simulink library "lib_dGrid"  (R2023b)
settings: Solver=VariableStepAuto  StartTime=0.0  StopTime=10.0  RelTol=1e-3
values from neighbouring files (symbols this model uses):
  C_PM = 10e-3    (= 0.01)    [my_MMC_param.m]
  Cbase = 1/Zbase/wb    (= 3.10849498226e-05)    [my_MMC_param.m]
  f0 = 50/fb    (= 1)    [my_MMC_param.m]
  Fn_filter = 1000    [my_MMC_param.m]
  Fnom = 50    [my_MMC_param.m]
  GFL_APC = 1    [Analysis_Main.m]    (also in initSimu.m; my_MMC_param.m)
  GFL_DVC = 2    [Analysis_Main.m]    (also in initSimu.m; my_MMC_param.m)
  GFM_APC = 3; (values programmed in EMT models)    [Analysis_Main.m]    (also in initSimu.m; my_MMC_param.m = 3)
  GFM_VF = 0    [my_MMC_param.m]
  Ibase = 2*Sbase/(3*Ubase)    [my_MMC_param.m]
  Idcb = Sbase/Udcb    [my_MMC_param.m]
  Ki_Iccsc = 5.15    [my_MMC_param.m]
  Ki_Ireg = CCCTRL.CC.ki    [my_MMC_param.m]
  Ki_Izscc = 100    [my_MMC_param.m]
  Ki_PLL = 1/(CCCTRL.PLL.v0*CCCTRL.PLL.T^2)    [my_MMC_param.m]
  Ki_Preg = 1.0*10    (= 10)    [my_MMC_param.m]
  Ki_Qreg = 1.0*10    (= 10)    [my_MMC_param.m]
  Ki_VAC_GFL = 50    [my_MMC_param.m]
  Ki_VACreg = 10    [my_MMC_param.m]
  Ki_VDCreg = 10    [my_MMC_param.m]
  Ki_WtReg = Kp_WtReg / 0.025    (= 1600)    [my_MMC_param.m]
  Kp_Iccsc = 0.21    [my_MMC_param.m]
  Kp_Ireg = CCCTRL.CC.kp    [my_MMC_param.m]
  Kp_Izscc = 10    [my_MMC_param.m]
  Kp_PLL = 2/CCCTRL.PLL.v0/CCCTRL.PLL.T    [my_MMC_param.m]
  Kp_Preg = 0.5/3*1    (= 0.166666666667)    [my_MMC_param.m]
  Kp_Qreg = 0.5/3*1    (= 0.166666666667)    [my_MMC_param.m]
  Kp_VAC_GFL = 0.5    [my_MMC_param.m]
  Kp_VACreg = 0.01    [my_MMC_param.m]
  Kp_VDCreg = 1    [my_MMC_param.m]
  Kp_WtReg = 40    [my_MMC_param.m]
  Kpv_GFM = 1    [my_MMC_param.m]
  Kpwm = 0.5    [my_MMC_param.m]
  Larm = Larm_pu*(Zbase/wb)    (= 0.0488923985178)    [my_MMC_param.m]
  Lff = Larm_pu/2    (= 0.075)    [my_MMC_param.m]
  Limits_Ireg = [ 2.0  -2.0]    [my_MMC_param.m]
  Limits_Preg = [ 2, -2 ]    [my_MMC_param.m]
  Limits_Qreg = 2*[ 0.42, -0.42 ]    [my_MMC_param.m]
  Limits_VACreg = [ 1.3  -1.3]    [my_MMC_param.m]
  Limits_VDCreg = [ 2.0  -2.0]    [my_MMC_param.m]
  MMC1 = MMC    [Analysis_Main.m]    (also in initSimu.m)
  Nb_PM = 400    [my_MMC_param.m]
  PhaseDelay = 1.0*Ts_Control*2*pi*50    (= 0.0628318530718)    [my_MMC_param.m]
  Pnom = 1000e6    (= 1000000000)    [my_MMC_param.m]
  Rarm = Rarm_pu*Zbase    (= 0.1536)    [my_MMC_param.m]
  Slope_Pref = 0.5    [my_MMC_param.m]
  Slope_Qref = 0.5    [my_MMC_param.m]
  Slope_Vdc_ref = Vnom_dc/2    (= 320000)    [my_MMC_param.m]
  Tdeblock = 1.5    [my_MMC_param.m]
  Ton_CROSSreg = Ton_PQreg+3    (= 7)    [my_MMC_param.m]
  Ton_PQreg = 4    [my_MMC_param.m]
  Ton_VDCreg = 1.5    [my_MMC_param.m]
  Ts = Ts_Control    (= 0.0002)    [my_MMC_param.m]
  Ts_Control = Ts_Power*2    (= 0.0002)    [my_MMC_param.m]
  Ts_Power = 20e-6 * 5    (= 0.0001)    [my_MMC_param.m]
  Ubase = sqrt(2/3)*Vnom_sec    [my_MMC_param.m]
  Udcb = 2*Ubase    [my_MMC_param.m]
  Vc0_PM = 0    [my_MMC_param.m]
  Vnom_dc = 640e3    (= 640000)    [my_MMC_param.m]
  Vnom_sec = 320e3    (= 320000)    [my_MMC_param.m]
  wb = 2*pi*fb    (= 314.159265359)    [my_MMC_param.m]
  Wt_ref_pu = 0.5 * C_PM * (Vnom_dc/Nb_PM)^2 * Nb_PM * 6 / Pnom    (= 0.03072)    [my_MMC_param.m]
undefined symbols (not defined in the file or in its folder): ControlSampleTime, DiscIntNeverNeededParam, MMC, PLL, VSM
libraries: simulink x50, spsCurrentMeasurementLib x20, spsSecondOrderFilterLib x20, spsDiodeLib x12, spsControlledVoltageSourceLib x12, spsSeriesRLCBranchLib x10, spsFirstOrderFilterLib x9, spsVoltageMeasurementLib x8, spsMeanLib x7, FriedrichLibrary x6, $bdroot x6, powerlib_extras x4
(part 5 of 8)

== system lib_dGrid/MMC-configurable control modes/MMC Control/CCSC + ZSCC control/PI regulator with anti-windup D1 ==
  note: Anti-windup mechanism: Method of conditionnal integration
      |
      | The integration is suspended if saturation occurs and the
      | control error is of the same sign as the control signal.
      |
      | [1] L.Rundqwist, "Anti-Reset Windup for PID Controllers," Ph.D. Thesis TRFT-1033,
      | Departement of Automatic Control, Lund Institute of Technology, Lund, Sweeden, 1991.
  Error : Inport  SampleTime=Ts
  Compare To Zero : simulink/Logic and Bit Operations/Compare To Zero  relop=>  OutDataTypeStr=uint8  ZeroCross=off
  Compare To Zero1 : simulink/Logic and Bit Operations/Compare To Zero  relop=<  OutDataTypeStr=uint8  ZeroCross=off
  Constant : Constant  Value=0
  Constant1 : Constant  Value=UpperLimit
  Constant3 : Constant  Value=LowerLimit
  Discrete-Time Integrator : DiscreteIntegrator  IntegratorMethod=Integration: Trapezoidal  InitialCondition=Init  SampleTime=Ts  LimitOutput=on  UpperSaturationLimit=UpperLimit  LowerSaturationLimit=LowerLimit  ShowStatePort=on  ICPrevOutput=DiscIntNeverNeededParam  ICPrevScaledInput=DiscIntNeverNeededParam
  Kp4 : Gain  Gain=Kp  SaturateOnIntegerOverflow=on  SampleTime=Ts  OutDataTypeStr=Inherit: Same as input  ParamDataTypeStr=Inherit: Same as input
  Kp5 : Gain  Gain=Ki  SaturateOnIntegerOverflow=on  SampleTime=Ts  OutDataTypeStr=Inherit: Same as input  ParamDataTypeStr=Inherit: Same as input
  Logical Operator : Logic  AllPortsSameDT=off  OutDataTypeStr=boolean
  Logical Operator1 : Logic  AllPortsSameDT=off  OutDataTypeStr=boolean
  Logical Operator2 : Logic  Operator=OR  AllPortsSameDT=off  OutDataTypeStr=boolean
  Relational Operator : RelationalOperator  OutDataTypeStr=boolean  InputSameDT=off
  Relational Operator1 : RelationalOperator  Operator=<=  OutDataTypeStr=boolean  InputSameDT=off
  Saturation2 : Saturate  UpperLimit=UpperLimit  LowerLimit=LowerLimit  SampleTime=Ts
  Sum1 : Sum  InputSameDT=on  SaturateOnIntegerOverflow=on  SampleTime=Ts  OutDataTypeStr=Inherit: Same as first input
  Sum6 : Sum  InputSameDT=on  SaturateOnIntegerOverflow=on  SampleTime=Ts  OutDataTypeStr=Inherit: Same as first input
  Switch : Switch  Criteria=u2 > Threshold  SaturateOnIntegerOverflow=off  InputSameDT=off
  Zero-Order Hold : ZeroOrderHold  SampleTime=Ts
  Out : Outport  SampleTime=Ts  InitialOutput=0  VectorParamsAs1DForOutWhenUnconnected=off
  wires:
  Constant/1 -> Switch/1
  Zero-Order Hold/1 -> Sum1/2, Sum6/1
  Discrete-Time Integrator/State -> Sum1/1
  Sum1/1 -> Relational Operator1/1, Relational Operator/1
  Logical Operator2/1 -> Switch/2
  Relational Operator/1 -> Logical Operator/1  "UpperLimit_is_Reached"
  Relational Operator1/1 -> Logical Operator1/1  "LowerLimit_Is_Reached"
  Constant1/1 -> Relational Operator/2
  Constant3/1 -> Relational Operator1/2
  Compare To Zero/1 -> Logical Operator/2  "Error_is_positive"
  Logical Operator/1 -> Logical Operator2/1
  Logical Operator1/1 -> Logical Operator2/2
  Compare To Zero1/1 -> Logical Operator1/2  "Error_is_negative"
  Error/1 -> Compare To Zero1/1, Compare To Zero/1, Kp4/1, Kp5/1
  Sum6/1 -> Saturation2/1
  Kp4/1 -> Zero-Order Hold/1
  Discrete-Time Integrator/1 -> Sum6/2
  Saturation2/1 -> Out/1
  Switch/1 -> Discrete-Time Integrator/1
  Kp5/1 -> Switch/3

== system lib_dGrid/MMC-configurable control modes/MMC Control/CCSC + ZSCC control/PR control ==
  meas_icir_abc : Inport
  Demux2 : Demux  Outputs=3
  Mux2 : Mux  Inputs=3
  PR Controller : Subsystem  mask(PR Controller){kp=Kp_Iccsc, kr=Ki_Iccsc, f=100}
      mask prompts: kp "Proportional Gain (kp)"; kr "Resonant Gain (kr)"; f "Resonant Frequency (Hz)"
      mask help:
      | This block implements a Proportional Resonant Controller using transfer function kr*s / s^2+(2*pi*f)^2
      | It allows user to set the proportional gain (kp), resonant gain (kr) and resonant frequency in (Hz).
      |
      | Developed by Rodney Tan
      | Version 1.0 (Oct 2022)
      mask Display: disp('PR(s)');
  PR Controller1 : Subsystem  mask(PR Controller){kp=Kp_Iccsc, kr=Ki_Iccsc, f=100}
      mask prompts: kp "Proportional Gain (kp)"; kr "Resonant Gain (kr)"; f "Resonant Frequency (Hz)"
      mask help:
      | This block implements a Proportional Resonant Controller using transfer function kr*s / s^2+(2*pi*f)^2
      | It allows user to set the proportional gain (kp), resonant gain (kr) and resonant frequency in (Hz).
      |
      | Developed by Rodney Tan
      | Version 1.0 (Oct 2022)
      mask Display: disp('PR(s)');
  PR Controller2 : Subsystem  mask(PR Controller){kp=Kp_Iccsc, kr=Ki_Iccsc, f=100}
      mask prompts: kp "Proportional Gain (kp)"; kr "Resonant Gain (kr)"; f "Resonant Frequency (Hz)"
      mask help:
      | This block implements a Proportional Resonant Controller using transfer function kr*s / s^2+(2*pi*f)^2
      | It allows user to set the proportional gain (kp), resonant gain (kr) and resonant frequency in (Hz).
      |
      | Developed by Rodney Tan
      | Version 1.0 (Oct 2022)
      mask Display: disp('PR(s)');
  Out1 : Outport
  wires:
  PR Controller1/1(Out1) -> Mux2/2
  Demux2/2 -> PR Controller1/1(In1)
  Demux2/1 -> PR Controller/1(In1)
  meas_icir_abc/1 -> Demux2/1
  PR Controller2/1(Out1) -> Mux2/3
  Mux2/1 -> Out1/1
  PR Controller/1(Out1) -> Mux2/1
  Demux2/3 -> PR Controller2/1(In1)

== system lib_dGrid/MMC-configurable control modes/MMC Control/CCSC + ZSCC control/PhN->ab2 ==
  PhN : Inport
  AlphaBetaNull Transformation : Gain  Gain="[2/3   -1/3    -1/3;   0   1/sqrt(3) -1/sqrt(3); 1/3 1/3 1/3]"  Multiplication=Matrix(K*u) (u vector)
  ab0 : Outport  VectorParamsAs1DForOutWhenUnconnected=off
  wires:
  AlphaBetaNull Transformation/1 -> ab0/1
  PhN/1 -> AlphaBetaNull Transformation/1

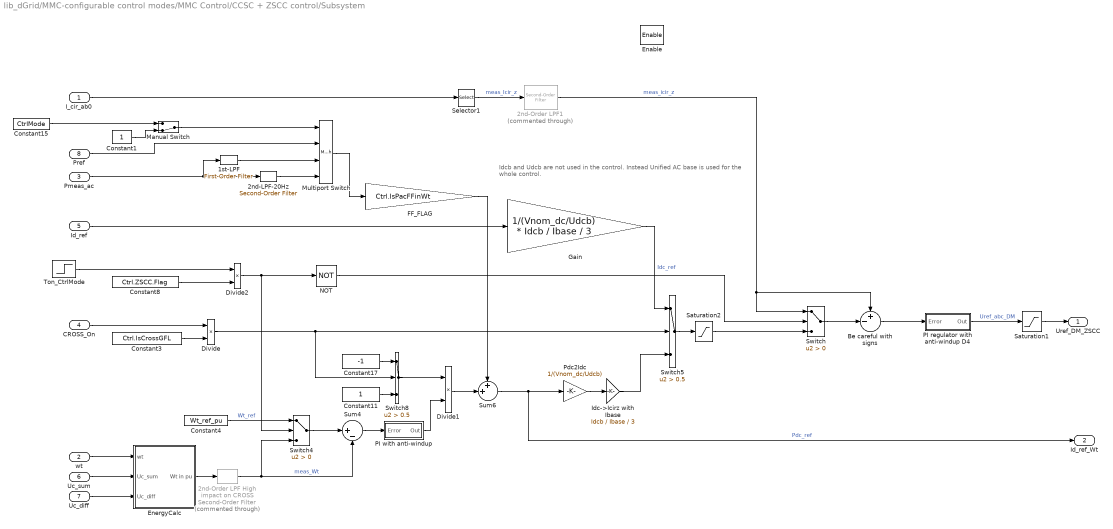
== system lib_dGrid/MMC-configurable control modes/MMC Control/CCSC + ZSCC control/Subsystem ==
  note: Idcb and Udcb are not used in the control. Instead
      | Unified AC base is used for the whole control.
  I_cir_ab0 : Inport
  wt : Inport  Port=2
  Pmeas_ac : Inport  Port=3
  CROSS_On : Inport  Port=4
  Id_ref : Inport  Port=5
  Uc_sum : Inport  Port=6
  Uc_diff : Inport  Port=7
  Pref : Inport  Port=8
  Enable : EnablePort  StatesWhenEnabling=reset
  1st-LPF : spsFirstOrderFilterLib/First-Order Filter  FilterType=Lowpass  Tc=1/(2*pi*20)  Ts=Ts_Control  Initialize=on  Vac_Init=[0, 0, 50]  Vdc_Init=0  PlotResponse=off  FreqRange="[0,  200,  1]"
  2nd-LPF-20Hz : spsSecondOrderFilterLib/Second-Order Filter  FilterType=Lowpass  Fo=Fn_filter/50  Zeta=Zeta_filter  Ts=Ts  Initialize=off  Vac_Init="[0,  0,  60]"  Vdc_Init=0  PlotResponse=off  FreqRange=[0, 500, 1]
      settings: LibrarySourceBlock=|
      | sps_lib/Control/Filters/Second-Order
      | Filter
  2nd-Order LPF1 : spsSecondOrderFilterLib/Second-Order Filter  Commented=through  FilterType=Lowpass  Fo=Fn_filter  Zeta=Zeta_filter  Ts=Ts  Initialize=off  Vac_Init="[0,  0,  60]"  Vdc_Init=0  PlotResponse=off  FreqRange=[0, 500, 1]
      settings: LibrarySourceBlock=|
      | sps_lib/Control/Filters/Second-Order
      | Filter
  2nd-Order LPF High impact on CROSS : spsSecondOrderFilterLib/Second-Order Filter  Commented=through  FilterType=Lowpass  Fo=Fn_filter  Zeta=Zeta_filter  Ts=Ts  Initialize=off  Vac_Init="[0,  0,  60]"  Vdc_Init=0  PlotResponse=off  FreqRange=[0, 500, 1]
      settings: LibrarySourceBlock=|
      | sps_lib/Control/Filters/Second-Order
      | Filter
  Be careful with signs : Sum  Inputs=+-|
  Constant1 : Constant
  Constant11 : Constant
  Constant15 : Constant  Value=CtrlMode
  Constant17 : Constant  Value=-1
  Constant3 : Constant  Value=Ctrl.IsCrossGFL
  Constant4 : Constant  Value=Wt_ref_pu
  Constant8 : Constant  Value=Ctrl.ZSCC.Flag
  Divide : Product  Inputs=**
  Divide1 : Product  Inputs=**
  Divide2 : Product  Inputs=**
  EnergyCalc : Subsystem
  FF_FLAG : Gain  Gain=Ctrl.IsPacFFinWt
  Gain : Gain  Gain=1/(Vnom_dc/Udcb) * Idcb / Ibase / 3
  Idc->Icirz with Ibase : Gain  Gain=Idcb / Ibase / 3
  Manual Switch : ManualSwitch  CurrentSetting=0
  Multiport Switch : MultiPortSwitch  SaturateOnIntegerOverflow=off
  NOT : Logic  Operator=NOT  IconShape=distinctive  AllPortsSameDT=off  OutDataTypeStr=boolean
  PI regulator with anti-windup D4 : Subsystem  DialogController=POWERSYS.PowerSysDialog  mask(Discrete PI Controller){Kp=Kp_Izscc, Ki=Ki_Izscc, Par_Limits=Limits_Ireg, Init=0, Ts=Ts_Control}
      mask prompts: Kp "Proportional gain (Kp):"; Ki "Integral gain (Ki):"; Par_Limits "Output limits: [ Upper   Lower ]"; Init "Output initial value:"; Ts "Sample time:"
      mask help: This block implements a discrete PI controller.
      mask init:
      | UpperLimit=Par_Limits(1);
      | LowerLimit=Par_Limits(2);
      | power_initmask();
      mask Help: This block is part of a subset of blocks in the Extras library that does not have documentation associated with it, other than the block mask description.
      mask Display: disp('PI');
  PI with anti-windup : Subsystem  DialogController=POWERSYS.PowerSysDialog  mask(Discrete PI Controller){Kp=Kp_WtReg, Ki=Ki_WtReg, Par_Limits=[1 -1], Init=0, Ts=Ts_Control}
      mask prompts: Kp "Proportional gain (Kp):"; Ki "Integral gain (Ki):"; Par_Limits "Output limits: [ Upper   Lower ]"; Init "Output initial value:"; Ts "Sample time:"
      mask help: This block implements a discrete PI controller.
      mask init:
      | UpperLimit=Par_Limits(1);
      | LowerLimit=Par_Limits(2);
      | power_initmask();
      mask Help: This block is part of a subset of blocks in the Extras library that does not have documentation associated with it, other than the block mask description.
      mask Display: disp('PI');
  Pdc2Idc : Gain  Gain=1/(Vnom_dc/Udcb)
  Saturation1 : Saturate  UpperLimit=0.8  LowerLimit=-0.8
  Saturation2 : Saturate  UpperLimit=1  LowerLimit=-1  SampleTime=Ts
  Selector1 : Selector  InputPortWidth=3  IndexOptions=Index vector (dialog)  Indices=3  OutputSizes=1
  Sum4 : Sum  Inputs=|+-
  Sum6 : Sum  Inputs=++|
  Switch : Switch  Criteria=u2 > Threshold  SaturateOnIntegerOverflow=off  InputSameDT=off
  Switch4 : Switch  Criteria=u2 > Threshold  SaturateOnIntegerOverflow=off  InputSameDT=off
  Switch5 : Switch  Criteria=u2 > Threshold  Threshold=0.5  SaturateOnIntegerOverflow=off  InputSameDT=off
  Switch8 : Switch  Criteria=u2 > Threshold  Threshold=0.5  SaturateOnIntegerOverflow=off  InputSameDT=off
  Ton_CtrlMode : Step  Time=Ton_PQreg  SampleTime=Ts
  Uref_DM_ZSCC : Outport
  Id_ref_Wt : Outport  Port=2
  wires:
  Sum6/1 -> Id_ref_Wt/1, Pdc2Idc/1  "Pdc_ref"
  PI regulator with anti-windup D4/1(Out) -> Saturation1/1  "Uref_abc_DM"
  2nd-Order LPF1/1 -> Be careful with signs/1, Switch/1  "meas_icir_z"
  Divide1/1 -> Sum6/2
  Pref/1 -> Multiport Switch/2
  FF_FLAG/1 -> Sum6/1
  2nd-Order LPF High impact on CROSS/1 -> Switch4/3, Sum4/2  "meas_Wt"
  I_cir_ab0/1 -> Selector1/1
  EnergyCalc/1(Wt in pu) -> 2nd-Order LPF High impact on CROSS/1
  Switch4/1 -> Sum4/1
  PI with anti-windup/1(Out) -> Divide1/2
  Selector1/1 -> 2nd-Order LPF1/1  "meas_Icir_z"
  Sum4/1 -> PI with anti-windup/1(Error)
  Pdc2Idc/1 -> Idc->Icirz with Ibase/1
  Pmeas_ac/1 -> 2nd-LPF-20Hz/1, 1st-LPF/1
  Switch/1 -> Be careful with signs/2
  Switch5/1 -> Saturation2/1
  1st-LPF/1 -> Multiport Switch/3
  NOT/1 -> Switch/2
  Gain/1 -> Switch5/1  "Idc_ref"
  Be careful with signs/1 -> PI regulator with anti-windup D4/1(Error)
  Uc_sum/1 -> EnergyCalc/2(Uc_sum)
  2nd-LPF-20Hz/1 -> Multiport Switch/4
  Divide2/1 -> Switch4/2, NOT/1
  Constant4/1 -> Switch4/1  "Wt_ref"
  Constant3/1 -> Divide/2
  Id_ref/1 -> Gain/1
  Saturation2/1 -> Switch/3
  Uc_diff/1 -> EnergyCalc/3(Uc_diff)
  Idc->Icirz with Ibase/1 -> Switch5/3
  Ton_CtrlMode/1 -> Divide2/1
  wt/1 -> EnergyCalc/1(wt)
  Saturation1/1 -> Uref_DM_ZSCC/1
  Multiport Switch/1 -> FF_FLAG/1
  Constant8/1 -> Divide2/2
  Constant17/1 -> Switch8/1
  Divide/1 -> Switch5/2, Switch8/2
  CROSS_On/1 -> Divide/1
  Constant11/1 -> Switch8/3
  Constant15/1 -> Manual Switch/1
  Switch8/1 -> Divide1/1
  Manual Switch/1 -> Multiport Switch/1
  Constant1/1 -> Manual Switch/2

== system lib_dGrid/MMC-configurable control modes/MMC Control/CCSC + ZSCC control/UCM ==
  note: Original implementation for modulation compensation
      |
      |
      |
      |
      |
      |
      |
      |
      | Equivalent to the control output divided by Vdc_pu
      | which can be calculated by Vdc/Vdc_base
      | where Vdc_base = 2 * Vbase with
      | Vbase = sqrt(2)/sqrt(3)*Vnom_sec
  Uref : Inport
  " (Hz)" : Constant  Commented=on  Value=Vnom_dc  SampleTime=Ts
  " (Hz)1" : Constant  Value=Vnom_dc  SampleTime=Ts
  ->pu : Gain  Gain=1/Udcb
  Avoid division by zero1 : Saturate  Commented=on  UpperLimit=Vnom_dc*1.25  LowerLimit=Vnom_dc*0.75
  Avoid division by zero2 : Saturate  UpperLimit=Vnom_dc*1.25  LowerLimit=Vnom_dc*0.75
  Divide : Product  Commented=on  Inputs=*/
  Divide1 : Product  Commented=on  Inputs=**
  Divide2 : Product  Inputs=*/
  Mean : spsMeanLib/Mean  Commented=on  Freq=Fnom/3  Vinit=Vnom_dc  Ts=Ts
  to-pu : Gain  Commented=on  Gain=1/(Vnom_dc/2*sqrt(3)/sqrt(2)/Vnom_sec)
  out : Outport
  wires:
  Divide1/1 -> to-pu/1
  " (Hz)"/1 -> Divide/1
  Divide/1 -> Divide1/2
  Divide2/1 -> out/1
  Avoid division by zero1/1 -> Divide/2
  ->pu/1 -> Divide2/2  "udc_pu"
  Uref/1 -> Divide2/1
  Avoid division by zero2/1 -> ->pu/1
  " (Hz)1"/1 -> Avoid division by zero2/1
  Mean/1 -> Avoid division by zero1/1

== system lib_dGrid/MMC-configurable control modes/MMC Control/CCSC + ZSCC control/ab0->dq0-faster1 ==
  ab0 : Inport
  w : Inport  Port=2
  Demux : Demux  Outputs=3
  Mux : Mux  Inputs=3
  Product{,1..3} (4 alike) : Product
  Subtract : Sum
  Subtract1 : Sum  Inputs=-+
  Trigonometric Function : Trigonometry  Operator=sincos
  dq0 : Outport  VectorParamsAs1DForOutWhenUnconnected=off
  wires:
  Subtract/1 -> Mux/1
  Subtract1/1 -> Mux/2
  Product3/1 -> Subtract1/2
  Product2/1 -> Subtract1/1
  Product1/1 -> Subtract/2
  Product/1 -> Subtract/1
  Trigonometric Function/1 -> Product1/1, Product2/1
  Trigonometric Function/2 -> Product3/1, Product/1
  Demux/2 -> Product3/2, Product1/2
  w/1 -> Trigonometric Function/1
  ab0/1 -> Demux/1
  Demux/1 -> Product/2, Product2/2
  Demux/3 -> Mux/3
  Mux/1 -> dq0/1

== system lib_dGrid/MMC-configurable control modes/MMC Control/CCSC + ZSCC control/dq0->ab0 phi ua=cos(phi)*ud-sin(phi)*uq ub=-sin(phi)*ud+cos(phi)*uq1 ==
  dq0 : Inport
  phi : Inport  Port=2
  Demux : Demux  Outputs=3
  Mux : Mux  Inputs=3
  Product{,1..3} (4 alike) : Product
  Subtract : Sum  Inputs=+-
  Subtract1 : Sum
  Trigonometric Function : Trigonometry  Operator=sincos
  "ab0 " : Outport  VectorParamsAs1DForOutWhenUnconnected=off
  wires:
  Subtract/1 -> Mux/1
  Subtract1/1 -> Mux/2
  Product3/1 -> Subtract1/2
  Product2/1 -> Subtract1/1
  Product1/1 -> Subtract/2
  Product/1 -> Subtract/1
  Trigonometric Function/1 -> Product2/1, Product1/1
  Trigonometric Function/2 -> Product3/1, Product/1
  Demux/2 -> Product3/2, Product1/2
  dq0/1 -> Demux/1
  Demux/1 -> Product/2, Product2/2
  Demux/3 -> Mux/3
  Mux/1 -> "ab0 "/1
  phi/1 -> Trigonometric Function/1

== system lib_dGrid/MMC-configurable control modes/MMC Control/Compensation Modes & AC//DC to Arm transform Number of inserted (Nin) and blocked (Nbl) modules/PWM ==
  In1 : Inport
  Add{,7..11} (6 alike) : Sum  Inputs=1
  Constant{7..10,12..13} (6 alike) : Constant  Value=0
  Demux1 : Demux  Outputs=6
  Mux{9..14} (6 alike) : Mux  Inputs=2
  Mux15 : Mux  Inputs=6
  PWM Gen1 : Subsystem  mask(PWM generator for half-bridge MMC){n=Nb_PM, Fc=Fnom*3.37, Ts=Ts_Power}
      mask prompts: n "Number of half-bridges"; Fc "Carriers frequency (Hz)"; Ts "Sample time (s)"
      mask init:
      | Tc=1/Fc;
      |         Pc= [ 0:360/n:360-360/n]*pi/180;
      |         Offset=Pc/(2*pi);
      |         Offset_Cr=Pc/(2*pi)*Tc;
      |         p=0;
      |         for m=1:2:2*n
      |             p=p+1;
      |             SelectPulsesPS(m)=p;
      |             SelectPulsesPS(m+1)=p+n;
      |         end
  PWM Gen2 : Subsystem  mask(PWM generator for half-bridge MMC){n=Nb_PM, Fc=Fnom*3.37, Ts=Ts_Power}
      mask prompts: n "Number of half-bridges"; Fc "Carriers frequency (Hz)"; Ts "Sample time (s)"
      mask init: same as lib_dGrid/MMC-configurable control modes/MMC Control/Compensation Modes & AC//DC to Arm transform Number of inserted (Nin) and blocked (Nbl) modules/PWM/PWM Gen1
  PWM Gen3 : Subsystem  mask(PWM generator for half-bridge MMC){n=Nb_PM, Fc=Fnom*3.37, Ts=Ts_Power}
      mask prompts: n "Number of half-bridges"; Fc "Carriers frequency (Hz)"; Ts "Sample time (s)"
      mask init: same as lib_dGrid/MMC-configurable control modes/MMC Control/Compensation Modes & AC//DC to Arm transform Number of inserted (Nin) and blocked (Nbl) modules/PWM/PWM Gen1
  PWM Gen4 : Subsystem  mask(PWM generator for half-bridge MMC){n=Nb_PM, Fc=Fnom*3.37, Ts=Ts_Power}
      mask prompts: n "Number of half-bridges"; Fc "Carriers frequency (Hz)"; Ts "Sample time (s)"
      mask init: same as lib_dGrid/MMC-configurable control modes/MMC Control/Compensation Modes & AC//DC to Arm transform Number of inserted (Nin) and blocked (Nbl) modules/PWM/PWM Gen1
  PWM Gen5 : Subsystem  mask(PWM generator for half-bridge MMC){n=Nb_PM, Fc=Fnom*3.37, Ts=Ts_Power}
      mask prompts: n "Number of half-bridges"; Fc "Carriers frequency (Hz)"; Ts "Sample time (s)"
      mask init: same as lib_dGrid/MMC-configurable control modes/MMC Control/Compensation Modes & AC//DC to Arm transform Number of inserted (Nin) and blocked (Nbl) modules/PWM/PWM Gen1
  PWM Gen6 : Subsystem  mask(PWM generator for half-bridge MMC){n=Nb_PM, Fc=Fnom*3.37, Ts=Ts_Power}
      mask prompts: n "Number of half-bridges"; Fc "Carriers frequency (Hz)"; Ts "Sample time (s)"
      mask init: same as lib_dGrid/MMC-configurable control modes/MMC Control/Compensation Modes & AC//DC to Arm transform Number of inserted (Nin) and blocked (Nbl) modules/PWM/PWM Gen1
  Selector{1..6} (6 alike) : Selector  InputPortWidth=2*Nb_PM  IndexOptions=Index vector (dialog)  Indices=[1:2:2*Nb_PM-1]  OutputSizes=1
  Terminator{,1..5} (6 alike) : Terminator
  Out1 : Outport
  wires:
  Selector1/1 -> Add/1
  PWM Gen2/2(Cr) -> Terminator/1
  Selector2/1 -> Add7/1
  Mux10/1 -> Mux15/2
  Demux1/5 -> PWM Gen5/1(Uref)
  PWM Gen1/2(Cr) -> Terminator5/1
  Constant7/1 -> Mux9/2
  Mux9/1 -> Mux15/1
  PWM Gen4/2(Cr) -> Terminator4/1
  Selector3/1 -> Add9/1
  PWM Gen6/2(Cr) -> Terminator3/1
  Constant10/1 -> Mux12/2
  Constant12/1 -> Mux13/2
  PWM Gen3/1(P) -> Selector4/1
  PWM Gen2/1(P) -> Selector2/1
  Add9/1 -> Mux12/1
  Selector6/1 -> Add11/1
  Mux14/1 -> Mux15/6
  Mux12/1 -> Mux15/4
  PWM Gen5/1(P) -> Selector5/1
  Mux15/1 -> Out1/1
  Mux13/1 -> Mux15/5
  Demux1/6 -> PWM Gen6/1(Uref)
  Constant9/1 -> Mux11/2
  Constant8/1 -> Mux10/2
  Demux1/2 -> PWM Gen2/1(Uref)
  Mux11/1 -> Mux15/3
  Demux1/4 -> PWM Gen4/1(Uref)
  Demux1/3 -> PWM Gen3/1(Uref)
  Constant13/1 -> Mux14/2
  Add11/1 -> Mux14/1
  Add8/1 -> Mux11/1
  PWM Gen6/1(P) -> Selector6/1
  Selector4/1 -> Add8/1
  PWM Gen4/1(P) -> Selector3/1
  Add10/1 -> Mux13/1
  Demux1/1 -> PWM Gen1/1(Uref)
  PWM Gen1/1(P) -> Selector1/1
  Selector5/1 -> Add10/1
  PWM Gen3/2(Cr) -> Terminator1/1
  Add/1 -> Mux9/1
  In1/1 -> Demux1/1
  PWM Gen5/2(Cr) -> Terminator2/1
  Add7/1 -> Mux10/1

== system lib_dGrid/MMC-configurable control modes/MMC Control/Current Regulator/Modulation Gain ==
  note: Original implementation for modulation compensation
      |
      |
      |
      |
      |
      |
      |
      |
      | Equivalent to the control output divided by Vdc_pu
      | which can be calculated by Vdc/Vdc_base
      | where Vdc_base = 2 * Vbase with
      | Vbase = sqrt(2)/sqrt(3)*Vnom_sec
  Uref : Inport
  " (Hz)" : Constant  Commented=on  Value=Vnom_dc  SampleTime=Ts
  " (Hz)1" : Constant  Value=Vnom_dc  SampleTime=Ts
  ->pu : Gain  Gain=1/Udcb
  Avoid division by zero1 : Saturate  Commented=on  UpperLimit=Vnom_dc*1.25  LowerLimit=Vnom_dc*0.75
  Avoid division by zero2 : Saturate  UpperLimit=Vnom_dc*1.25  LowerLimit=Vnom_dc*0.75
  Divide : Product  Commented=on  Inputs=*/
  Divide1 : Product  Commented=on  Inputs=**
  Divide2 : Product  Inputs=*/
  Mean : spsMeanLib/Mean  Commented=on  Freq=Fnom/3  Vinit=Vnom_dc  Ts=Ts
  to-pu : Gain  Commented=on  Gain=1/(Vnom_dc/2*sqrt(3)/sqrt(2)/Vnom_sec)
  out : Outport
  wires:
  Divide1/1 -> to-pu/1
  " (Hz)"/1 -> Divide/1
  Divide/1 -> Divide1/2
  Divide2/1 -> out/1
  Avoid division by zero1/1 -> Divide/2
  ->pu/1 -> Divide2/2  "udc_pu"
  Avoid division by zero2/1 -> ->pu/1
  " (Hz)1"/1 -> Avoid division by zero2/1
  Mean/1 -> Avoid division by zero1/1
  Uref/1 -> Divide2/1

== system lib_dGrid/MMC-configurable control modes/MMC Control/Current Regulator/PI regulator with anti-windup D ==
  note: Anti-windup mechanism: Method of conditionnal integration
      |
      | The integration is suspended if saturation occurs and the
      | control error is of the same sign as the control signal.
      |
      | [1] L.Rundqwist, "Anti-Reset Windup for PID Controllers," Ph.D. Thesis TRFT-1033,
      | Departement of Automatic Control, Lund Institute of Technology, Lund, Sweeden, 1991.
  Error : Inport  SampleTime=Ts
  Compare To Zero : simulink/Logic and Bit Operations/Compare To Zero  relop=>  OutDataTypeStr=uint8  ZeroCross=off
  Compare To Zero1 : simulink/Logic and Bit Operations/Compare To Zero  relop=<  OutDataTypeStr=uint8  ZeroCross=off
  Constant : Constant  Value=0
  Constant1 : Constant  Value=UpperLimit
  Constant3 : Constant  Value=LowerLimit
  Discrete-Time Integrator : DiscreteIntegrator  IntegratorMethod=Integration: Trapezoidal  InitialCondition=Init  SampleTime=Ts  LimitOutput=on  UpperSaturationLimit=UpperLimit  LowerSaturationLimit=LowerLimit  ShowStatePort=on  ICPrevOutput=DiscIntNeverNeededParam  ICPrevScaledInput=DiscIntNeverNeededParam
  Kp4 : Gain  Gain=Kp  SaturateOnIntegerOverflow=on  SampleTime=Ts  OutDataTypeStr=Inherit: Same as input  ParamDataTypeStr=Inherit: Same as input
  Kp5 : Gain  Gain=Ki  SaturateOnIntegerOverflow=on  SampleTime=Ts  OutDataTypeStr=Inherit: Same as input  ParamDataTypeStr=Inherit: Same as input
  Logical Operator : Logic  AllPortsSameDT=off  OutDataTypeStr=boolean
  Logical Operator1 : Logic  AllPortsSameDT=off  OutDataTypeStr=boolean
  Logical Operator2 : Logic  Operator=OR  AllPortsSameDT=off  OutDataTypeStr=boolean
  Relational Operator : RelationalOperator  OutDataTypeStr=boolean  InputSameDT=off
  Relational Operator1 : RelationalOperator  Operator=<=  OutDataTypeStr=boolean  InputSameDT=off
  Saturation2 : Saturate  UpperLimit=UpperLimit  LowerLimit=LowerLimit  SampleTime=Ts
  Sum1 : Sum  InputSameDT=on  SaturateOnIntegerOverflow=on  SampleTime=Ts  OutDataTypeStr=Inherit: Same as first input
  Sum6 : Sum  InputSameDT=on  SaturateOnIntegerOverflow=on  SampleTime=Ts  OutDataTypeStr=Inherit: Same as first input
  Switch : Switch  Criteria=u2 > Threshold  SaturateOnIntegerOverflow=off  InputSameDT=off
  Zero-Order Hold : ZeroOrderHold  Commented=through  SampleTime=Ts
  Out : Outport  SampleTime=Ts  InitialOutput=0  VectorParamsAs1DForOutWhenUnconnected=off
  wires:
  Constant/1 -> Switch/1
  Zero-Order Hold/1 -> Sum1/2, Sum6/1
  Discrete-Time Integrator/State -> Sum1/1
  Sum1/1 -> Relational Operator1/1, Relational Operator/1
  Logical Operator2/1 -> Switch/2
  Relational Operator/1 -> Logical Operator/1  "UpperLimit_is_Reached"
  Relational Operator1/1 -> Logical Operator1/1  "LowerLimit_Is_Reached"
  Constant1/1 -> Relational Operator/2
  Constant3/1 -> Relational Operator1/2
  Compare To Zero/1 -> Logical Operator/2  "Error_is_positive"
  Logical Operator/1 -> Logical Operator2/1
  Logical Operator1/1 -> Logical Operator2/2
  Compare To Zero1/1 -> Logical Operator1/2  "Error_is_negative"
  Error/1 -> Compare To Zero1/1, Compare To Zero/1, Kp4/1, Kp5/1
  Sum6/1 -> Saturation2/1
  Kp4/1 -> Zero-Order Hold/1
  Discrete-Time Integrator/1 -> Sum6/2
  Saturation2/1 -> Out/1
  Switch/1 -> Discrete-Time Integrator/1
  Kp5/1 -> Switch/3

== system lib_dGrid/MMC-configurable control modes/MMC Control/Current Regulator/PI regulator with anti-windup D1 ==
  note: Anti-windup mechanism: Method of conditionnal integration
      |
      | The integration is suspended if saturation occurs and the
      | control error is of the same sign as the control signal.
      |
      | [1] L.Rundqwist, "Anti-Reset Windup for PID Controllers," Ph.D. Thesis TRFT-1033,
      | Departement of Automatic Control, Lund Institute of Technology, Lund, Sweeden, 1991.
  Error : Inport  SampleTime=Ts
  Compare To Zero : simulink/Logic and Bit Operations/Compare To Zero  relop=>  OutDataTypeStr=uint8  ZeroCross=off
  Compare To Zero1 : simulink/Logic and Bit Operations/Compare To Zero  relop=<  OutDataTypeStr=uint8  ZeroCross=off
  Constant : Constant  Value=0
  Constant1 : Constant  Value=UpperLimit
  Constant3 : Constant  Value=LowerLimit
  Discrete-Time Integrator : DiscreteIntegrator  IntegratorMethod=Integration: Trapezoidal  InitialCondition=Init  SampleTime=Ts  LimitOutput=on  UpperSaturationLimit=UpperLimit  LowerSaturationLimit=LowerLimit  ShowStatePort=on  ICPrevOutput=DiscIntNeverNeededParam  ICPrevScaledInput=DiscIntNeverNeededParam
  Kp4 : Gain  Gain=Kp  SaturateOnIntegerOverflow=on  SampleTime=Ts  OutDataTypeStr=Inherit: Same as input  ParamDataTypeStr=Inherit: Same as input
  Kp5 : Gain  Gain=Ki  SaturateOnIntegerOverflow=on  SampleTime=Ts  OutDataTypeStr=Inherit: Same as input  ParamDataTypeStr=Inherit: Same as input
  Logical Operator : Logic  AllPortsSameDT=off  OutDataTypeStr=boolean
  Logical Operator1 : Logic  AllPortsSameDT=off  OutDataTypeStr=boolean
  Logical Operator2 : Logic  Operator=OR  AllPortsSameDT=off  OutDataTypeStr=boolean
  Relational Operator : RelationalOperator  OutDataTypeStr=boolean  InputSameDT=off
  Relational Operator1 : RelationalOperator  Operator=<=  OutDataTypeStr=boolean  InputSameDT=off
  Saturation2 : Saturate  UpperLimit=UpperLimit  LowerLimit=LowerLimit  SampleTime=Ts
  Sum1 : Sum  InputSameDT=on  SaturateOnIntegerOverflow=on  SampleTime=Ts  OutDataTypeStr=Inherit: Same as first input
  Sum6 : Sum  InputSameDT=on  SaturateOnIntegerOverflow=on  SampleTime=Ts  OutDataTypeStr=Inherit: Same as first input
  Switch : Switch  Criteria=u2 > Threshold  SaturateOnIntegerOverflow=off  InputSameDT=off
  Zero-Order Hold : ZeroOrderHold  SampleTime=Ts
  Out : Outport  SampleTime=Ts  InitialOutput=0  VectorParamsAs1DForOutWhenUnconnected=off
  wires:
  Constant/1 -> Switch/1
  Zero-Order Hold/1 -> Sum1/2, Sum6/1
  Discrete-Time Integrator/State -> Sum1/1
  Sum1/1 -> Relational Operator1/1, Relational Operator/1
  Logical Operator2/1 -> Switch/2
  Relational Operator/1 -> Logical Operator/1  "UpperLimit_is_Reached"
  Relational Operator1/1 -> Logical Operator1/1  "LowerLimit_Is_Reached"
  Constant1/1 -> Relational Operator/2
  Constant3/1 -> Relational Operator1/2
  Compare To Zero/1 -> Logical Operator/2  "Error_is_positive"
  Logical Operator/1 -> Logical Operator2/1
  Logical Operator1/1 -> Logical Operator2/2
  Compare To Zero1/1 -> Logical Operator1/2  "Error_is_negative"
  Error/1 -> Compare To Zero1/1, Compare To Zero/1, Kp4/1, Kp5/1
  Sum6/1 -> Saturation2/1
  Kp4/1 -> Zero-Order Hold/1
  Discrete-Time Integrator/1 -> Sum6/2
  Saturation2/1 -> Out/1
  Switch/1 -> Discrete-Time Integrator/1
  Kp5/1 -> Switch/3

== system lib_dGrid/MMC-configurable control modes/MMC Control/Current Regulator/PI regulator with anti-windup D2 ==
  note: Anti-windup mechanism: Method of conditionnal integration
      |
      | The integration is suspended if saturation occurs and the
      | control error is of the same sign as the control signal.
      |
      | [1] L.Rundqwist, "Anti-Reset Windup for PID Controllers," Ph.D. Thesis TRFT-1033,
      | Departement of Automatic Control, Lund Institute of Technology, Lund, Sweeden, 1991.
  Error : Inport  SampleTime=Ts
  Compare To Zero : simulink/Logic and Bit Operations/Compare To Zero  relop=>  OutDataTypeStr=uint8  ZeroCross=off
  Compare To Zero1 : simulink/Logic and Bit Operations/Compare To Zero  relop=<  OutDataTypeStr=uint8  ZeroCross=off
  Constant : Constant  Value=0
  Constant1 : Constant  Value=UpperLimit
  Constant3 : Constant  Value=LowerLimit
  Discrete-Time Integrator : DiscreteIntegrator  IntegratorMethod=Integration: Trapezoidal  InitialCondition=Init  SampleTime=Ts  LimitOutput=on  UpperSaturationLimit=UpperLimit  LowerSaturationLimit=LowerLimit  ShowStatePort=on  ICPrevOutput=DiscIntNeverNeededParam  ICPrevScaledInput=DiscIntNeverNeededParam
  Kp4 : Gain  Gain=Kp  SaturateOnIntegerOverflow=on  SampleTime=Ts  OutDataTypeStr=Inherit: Same as input  ParamDataTypeStr=Inherit: Same as input
  Kp5 : Gain  Gain=Ki  SaturateOnIntegerOverflow=on  SampleTime=Ts  OutDataTypeStr=Inherit: Same as input  ParamDataTypeStr=Inherit: Same as input
  Logical Operator : Logic  AllPortsSameDT=off  OutDataTypeStr=boolean
  Logical Operator1 : Logic  AllPortsSameDT=off  OutDataTypeStr=boolean
  Logical Operator2 : Logic  Operator=OR  AllPortsSameDT=off  OutDataTypeStr=boolean
  Relational Operator : RelationalOperator  OutDataTypeStr=boolean  InputSameDT=off
  Relational Operator1 : RelationalOperator  Operator=<=  OutDataTypeStr=boolean  InputSameDT=off
  Saturation2 : Saturate  UpperLimit=UpperLimit  LowerLimit=LowerLimit  SampleTime=Ts
  Sum1 : Sum  InputSameDT=on  SaturateOnIntegerOverflow=on  SampleTime=Ts  OutDataTypeStr=Inherit: Same as first input
  Sum6 : Sum  InputSameDT=on  SaturateOnIntegerOverflow=on  SampleTime=Ts  OutDataTypeStr=Inherit: Same as first input
  Switch : Switch  Criteria=u2 > Threshold  SaturateOnIntegerOverflow=off  InputSameDT=off
  Zero-Order Hold : ZeroOrderHold  SampleTime=Ts
  Out : Outport  SampleTime=Ts  InitialOutput=0  VectorParamsAs1DForOutWhenUnconnected=off
  wires:
  Constant/1 -> Switch/1
  Zero-Order Hold/1 -> Sum1/2, Sum6/1
  Discrete-Time Integrator/State -> Sum1/1
  Sum1/1 -> Relational Operator1/1, Relational Operator/1
  Logical Operator2/1 -> Switch/2
  Relational Operator/1 -> Logical Operator/1  "UpperLimit_is_Reached"
  Relational Operator1/1 -> Logical Operator1/1  "LowerLimit_Is_Reached"
  Constant1/1 -> Relational Operator/2
  Constant3/1 -> Relational Operator1/2
  Compare To Zero/1 -> Logical Operator/2  "Error_is_positive"
  Logical Operator/1 -> Logical Operator2/1
  Logical Operator1/1 -> Logical Operator2/2
  Compare To Zero1/1 -> Logical Operator1/2  "Error_is_negative"
  Error/1 -> Compare To Zero1/1, Compare To Zero/1, Kp4/1, Kp5/1
  Sum6/1 -> Saturation2/1
  Kp4/1 -> Zero-Order Hold/1
  Discrete-Time Integrator/1 -> Sum6/2
  Saturation2/1 -> Out/1
  Switch/1 -> Discrete-Time Integrator/1
  Kp5/1 -> Switch/3

== system lib_dGrid/MMC-configurable control modes/MMC Control/Current Regulator/PI regulator with anti-windup Q ==
  note: Anti-windup mechanism: Method of conditionnal integration
      |
      | The integration is suspended if saturation occurs and the
      | control error is of the same sign as the control signal.
      |
      | [1] L.Rundqwist, "Anti-Reset Windup for PID Controllers," Ph.D. Thesis TRFT-1033,
      | Departement of Automatic Control, Lund Institute of Technology, Lund, Sweeden, 1991.
  Error : Inport  SampleTime=Ts
  Compare To Zero : simulink/Logic and Bit Operations/Compare To Zero  relop=>  OutDataTypeStr=uint8  ZeroCross=off
  Compare To Zero1 : simulink/Logic and Bit Operations/Compare To Zero  relop=<  OutDataTypeStr=uint8  ZeroCross=off
  Constant : Constant  Value=0
  Constant1 : Constant  Value=UpperLimit
  Constant3 : Constant  Value=LowerLimit
  Discrete-Time Integrator : DiscreteIntegrator  IntegratorMethod=Integration: Trapezoidal  InitialCondition=Init  SampleTime=Ts  LimitOutput=on  UpperSaturationLimit=UpperLimit  LowerSaturationLimit=LowerLimit  ShowStatePort=on  ICPrevOutput=DiscIntNeverNeededParam  ICPrevScaledInput=DiscIntNeverNeededParam
  Kp4 : Gain  Gain=Kp  SaturateOnIntegerOverflow=on  SampleTime=Ts  OutDataTypeStr=Inherit: Same as input  ParamDataTypeStr=Inherit: Same as input
  Kp5 : Gain  Gain=Ki  SaturateOnIntegerOverflow=on  SampleTime=Ts  OutDataTypeStr=Inherit: Same as input  ParamDataTypeStr=Inherit: Same as input
  Logical Operator : Logic  AllPortsSameDT=off  OutDataTypeStr=boolean
  Logical Operator1 : Logic  AllPortsSameDT=off  OutDataTypeStr=boolean
  Logical Operator2 : Logic  Operator=OR  AllPortsSameDT=off  OutDataTypeStr=boolean
  Relational Operator : RelationalOperator  OutDataTypeStr=boolean  InputSameDT=off
  Relational Operator1 : RelationalOperator  Operator=<=  OutDataTypeStr=boolean  InputSameDT=off
  Saturation2 : Saturate  UpperLimit=UpperLimit  LowerLimit=LowerLimit  SampleTime=Ts
  Sum1 : Sum  InputSameDT=on  SaturateOnIntegerOverflow=on  SampleTime=Ts  OutDataTypeStr=Inherit: Same as first input
  Sum6 : Sum  InputSameDT=on  SaturateOnIntegerOverflow=on  SampleTime=Ts  OutDataTypeStr=Inherit: Same as first input
  Switch : Switch  Criteria=u2 > Threshold  SaturateOnIntegerOverflow=off  InputSameDT=off
  Zero-Order Hold : ZeroOrderHold  SampleTime=Ts
  Out : Outport  SampleTime=Ts  InitialOutput=0  VectorParamsAs1DForOutWhenUnconnected=off
  wires:
  Kp5/1 -> Switch/3
  Switch/1 -> Discrete-Time Integrator/1
  Saturation2/1 -> Out/1
  Discrete-Time Integrator/1 -> Sum6/2
  Kp4/1 -> Zero-Order Hold/1
  Sum6/1 -> Saturation2/1
  Error/1 -> Kp5/1, Kp4/1, Compare To Zero/1, Compare To Zero1/1
  Compare To Zero1/1 -> Logical Operator1/2  "Error_is_negative"
  Logical Operator1/1 -> Logical Operator2/2
  Logical Operator/1 -> Logical Operator2/1
  Compare To Zero/1 -> Logical Operator/2  "Error_is_positive"
  Constant3/1 -> Relational Operator1/2
  Constant1/1 -> Relational Operator/2
  Relational Operator1/1 -> Logical Operator1/1  "LowerLimit_Is_Reached"
  Relational Operator/1 -> Logical Operator/1  "UpperLimit_is_Reached"
  Logical Operator2/1 -> Switch/2
  Sum1/1 -> Relational Operator/1, Relational Operator1/1
  Discrete-Time Integrator/State -> Sum1/1
  Zero-Order Hold/1 -> Sum6/1, Sum1/2
  Constant/1 -> Switch/1

== system lib_dGrid/MMC-configurable control modes/MMC Control/GFL//GFM Switching & Modulation (UCM // DM) & dq0 ->abc/  ==
  AB0 : Inport
  Gain : Gain  Gain=1/2
  ab0->abc : Gain  Gain=[2 0 2; -1 sqrt(3) 2; -1 -sqrt(3) 2]  Multiplication=Matrix(K*u) (u vector)
  abc : Outport  SampleTime=Ts_Control  VectorParamsAs1DForOutWhenUnconnected=off
  wires:
  ab0->abc/1 -> abc/1
  AB0/1 -> Gain/1
  Gain/1 -> ab0->abc/1

== system lib_dGrid/MMC-configurable control modes/MMC Control/GFL//GFM Switching & Modulation (UCM // DM) & dq0 ->abc/dq0->ab0 phi ua=cos(phi)*ud-sin(phi)*uq ub=-sin(phi)*ud+cos(phi)*uq ==
  dq0 : Inport
  phi : Inport  Port=2
  Demux : Demux  Outputs=3
  Mux : Mux  Inputs=3
  Product{,1..3} (4 alike) : Product
  Subtract : Sum  Inputs=+-
  Subtract1 : Sum
  Trigonometric Function : Trigonometry  Operator=sincos
  "ab0 " : Outport  VectorParamsAs1DForOutWhenUnconnected=off
  wires:
  Subtract/1 -> Mux/1
  Subtract1/1 -> Mux/2
  Product3/1 -> Subtract1/2
  Product2/1 -> Subtract1/1
  Product1/1 -> Subtract/2
  Product/1 -> Subtract/1
  Trigonometric Function/1 -> Product2/1, Product1/1
  Trigonometric Function/2 -> Product3/1, Product/1
  Demux/2 -> Product3/2, Product1/2
  dq0/1 -> Demux/1
  Demux/1 -> Product/2, Product2/2
  Demux/3 -> Mux/3
  Mux/1 -> "ab0 "/1
  phi/1 -> Trigonometric Function/1

== system lib_dGrid/MMC-configurable control modes/MMC Control/PLL, Measurements and Transformation/PhN->ab1 ==
  PhN : Inport
  AlphaBetaNull Transformation : Gain  Gain="[2/3   -1/3    -1/3;   0   1/sqrt(3) -1/sqrt(3); 1/3 1/3 1/3]"  Multiplication=Matrix(K*u) (u vector)
  ab0 : Outport  VectorParamsAs1DForOutWhenUnconnected=off
  wires:
  AlphaBetaNull Transformation/1 -> ab0/1
  PhN/1 -> AlphaBetaNull Transformation/1

== system lib_dGrid/MMC-configurable control modes/MMC Control/PLL, Measurements and Transformation/PhN->ab2 ==
  PhN : Inport
  AlphaBetaNull Transformation : Gain  Gain="[2/3   -1/3    -1/3;   0   1/sqrt(3) -1/sqrt(3); 1/3 1/3 1/3]"  Multiplication=Matrix(K*u) (u vector)
  ab0 : Outport  VectorParamsAs1DForOutWhenUnconnected=off
  wires:
  AlphaBetaNull Transformation/1 -> ab0/1
  PhN/1 -> AlphaBetaNull Transformation/1

== system lib_dGrid/MMC-configurable control modes/MMC Control/PLL, Measurements and Transformation/Symmetrical PLL ==
  Vabc_PhN : Inport
  Add1 : Sum  Inputs=+-
  Add2 : Sum  Commented=on  Inputs=+-
  Add3 : Sum  Commented=on  Inputs=+-
  Angle Integrator [SI] : Subsystem  AncestorBlock=FriedrichLibrary/Discrete Stuff/Angle Integrator [SI]  mask{Ts=Ts}
      mask prompts: Ts "SampleTime"
      mask DialogControl DescGroupVar Prompt: Angle Integrator [SI]
      mask DialogControl DescTextVar Prompt: Discrete Integrator for omega, resetting every 2*pi.
  Constant1 : Constant  Commented=on  Value=2*pi
  Constant2 : Constant  Value=2*pi*f0*50
  Demux1 : Demux  Outputs=2
  Integrator (discrete)1 : DiscreteIntegrator  IntegratorMethod=Integration: Backward Euler  gainval=1  InitialConditionSource=external  SampleTime=Ts_Control  ICPrevOutput=DiscIntNeverNeededParam  ICPrevScaledInput=DiscIntNeverNeededParam
  Integrator (discrete)2 : DiscreteIntegrator  Commented=on  IntegratorMethod=Integration: Backward Euler  gainval=1  InitialConditionSource=external  SampleTime=Ts_Control  ICPrevOutput=DiscIntNeverNeededParam  ICPrevScaledInput=DiscIntNeverNeededParam
  Mean : spsMeanLib/Mean  Commented=on  Freq=0.05  Vinit=2*pi*50  Ts=Ts_Power
  PhN->ab0 : Subsystem  AncestorBlock=FriedrichLibrary/Transformations/PhN->ab0
      mask Display:
      | plot([0 1], [0,1])
      | plot([0.1 0.25 0.4 0.25 0.25], [0.5 0.6 0.5 0.6 0.8]) % Stern
      | text(0.05,1,'PhN','VerticalAlignment','Top')
      | text(0.55, 0.3,'\alpha\beta0','texmode','on')
  Rem : Math  Commented=on  Operator=rem
  Scope3 : Scope  Commented=on  NumInputPorts=2
  Selector : Selector  InputPortWidth=3  IndexOptions=Index vector (dialog)  Indices=2  OutputSizes=1
  Selector1 : Selector  InputPortWidth=3  IndexOptions=Index vector (dialog)  Indices=[2 1]  OutputSizes=1
  Trigonometric Function1 : Trigonometry  Operator=atan2
  ab0->dq0-faster : Subsystem  AncestorBlock=FriedrichLibrary/Transformations/ab0->dq0-faster
      mask Display:
      | plot([0 1], [0,1])
      | text(0.05,0.8,'\alpha\beta0','texmode','on')
      | text(1, 0.5,'dq0','HorizontalAlignment','right')
      | text(0.05,0.3,'\phi','texmode','on')
  discrete PID : Subsystem  AncestorBlock=FriedrichLibrary/Discrete Stuff/discrete PID  mask{Kp=Kp_PLL, Ki=Ki_PLL, Kd=Kd_PLL, Ts=Ts_Control, x_init=2*pi*50}
      mask prompts: Kp "Proportional Gain"; Ki "Integral Gain"; Kd "Differential Gain"; Ts "SampleTime"; x_init "Initial Condition"
  "omega -> f" : Gain  Gain=1/2/pi
  f : Outport  VectorParamsAs1DForOutWhenUnconnected=off
  phi : Outport  Port=2  VectorParamsAs1DForOutWhenUnconnected=off
  meas_theta_ref : Outport  Port=3  VectorParamsAs1DForOutWhenUnconnected=off
  wires:
  ab0->dq0-faster/1(dq0) -> Selector/1
  Angle Integrator [SI]/1(phi) -> phi/1, ab0->dq0-faster/2(w)
  "omega -> f"/1 -> f/1
  Vabc_PhN/1 -> PhN->ab0/1(PhN)
  PhN->ab0/1(ab0) -> Selector1/1, ab0->dq0-faster/1(ab0)
  Selector1/1 -> Demux1/1
  Demux1/1 -> Trigonometric Function1/1
  Demux1/2 -> Trigonometric Function1/2
  Selector/1 -> discrete PID/1(e)
  Add2/1 -> Integrator (discrete)2/1  "d_w"
  Trigonometric Function1/1 -> Integrator (discrete)1/2, Integrator (discrete)2/2, Angle Integrator [SI]/2(phi0)
  Add1/1 -> Integrator (discrete)1/1  "d_w"
  Integrator (discrete)1/1 -> meas_theta_ref/1, Scope3/1  "meas_theta_ref"
  Constant2/1 -> Add1/2
  discrete PID/1(y) -> Angle Integrator [SI]/1(omega), "omega -> f"/1, Add1/1, Add2/1, Mean/1
  Add3/1 -> Scope3/2  "meas_theta"
  Constant1/1 -> Add3/2, Rem/2
  Mean/1 -> Add2/2
  Integrator (discrete)2/1 -> Rem/1
  Rem/1 -> Add3/1  "xxx"

== system lib_dGrid/MMC-configurable control modes/MMC Control/PLL, Measurements and Transformation/ab0->dq0-NS ==
  ab0 : Inport
  w : Inport  Port=2
  Demux : Demux  Outputs=3
  Gain : Gain  Commented=through  Gain=-1
  Mux : Mux  Inputs=3
  Product{,1..3} (4 alike) : Product
  Subtract : Sum
  Subtract1 : Sum  Inputs=-+
  Trigonometric Function : Trigonometry  Operator=sincos
  dq0 : Outport  VectorParamsAs1DForOutWhenUnconnected=off
  wires:
  Mux/1 -> dq0/1
  Demux/3 -> Mux/3
  Demux/1 -> Product2/2, Product/2
  ab0/1 -> Demux/1
  w/1 -> Trigonometric Function/1
  Demux/2 -> Product1/2, Product3/2
  Trigonometric Function/2 -> Product3/1, Product/1
  Trigonometric Function/1 -> Gain/1
  Product/1 -> Subtract/1
  Product1/1 -> Subtract/2
  Product2/1 -> Subtract1/1
  Product3/1 -> Subtract1/2
  Subtract1/1 -> Mux/2
  Subtract/1 -> Mux/1
  Gain/1 -> Product2/1, Product1/1

== system lib_dGrid/MMC-configurable control modes/MMC Control/PLL, Measurements and Transformation/ab0->dq0-faster ==
  ab0 : Inport
  w : Inport  Port=2
  Demux : Demux  Outputs=3
  Mux : Mux  Inputs=3
  Product{,1..3} (4 alike) : Product
  Subtract : Sum
  Subtract1 : Sum  Inputs=-+
  Trigonometric Function : Trigonometry  Operator=sincos
  dq0 : Outport  VectorParamsAs1DForOutWhenUnconnected=off
  wires:
  Subtract/1 -> Mux/1
  Subtract1/1 -> Mux/2
  Product3/1 -> Subtract1/2
  Product2/1 -> Subtract1/1
  Product1/1 -> Subtract/2
  Product/1 -> Subtract/1
  Trigonometric Function/1 -> Product1/1, Product2/1
  Trigonometric Function/2 -> Product3/1, Product/1
  Demux/2 -> Product3/2, Product1/2
  w/1 -> Trigonometric Function/1
  ab0/1 -> Demux/1
  Demux/1 -> Product/2, Product2/2
  Demux/3 -> Mux/3
  Mux/1 -> dq0/1

== system lib_dGrid/MMC-configurable control modes/MMC Control/PLL, Measurements and Transformation/ab0->dq0-faster1 ==
  ab0 : Inport
  w : Inport  Port=2
  Demux : Demux  Outputs=3
  Mux : Mux  Inputs=3
  Product{,1..3} (4 alike) : Product
  Subtract : Sum
  Subtract1 : Sum  Inputs=-+
  Trigonometric Function : Trigonometry  Operator=sincos
  dq0 : Outport  VectorParamsAs1DForOutWhenUnconnected=off
  wires:
  Subtract/1 -> Mux/1
  Subtract1/1 -> Mux/2
  Product3/1 -> Subtract1/2
  Product2/1 -> Subtract1/1
  Product1/1 -> Subtract/2
  Product/1 -> Subtract/1
  Trigonometric Function/1 -> Product1/1, Product2/1
  Trigonometric Function/2 -> Product3/1, Product/1
  Demux/2 -> Product3/2, Product1/2
  w/1 -> Trigonometric Function/1
  ab0/1 -> Demux/1
  Demux/1 -> Product/2, Product2/2
  Demux/3 -> Mux/3
  Mux/1 -> dq0/1

== system lib_dGrid/MMC-configurable control modes/MMC Control/PLL, Measurements and Transformation/from DDSRF-PLL ==
  ab0 : Inport
  w : Inport  Port=2
  Mux : Mux  Inputs=2
  PT1 as IIR : Subsystem  AncestorBlock=FriedrichLibrary/Discrete Stuff/PT1 as IIR  mask{K=1, tau=T1, Init=0, T=Ts_Control}
      mask prompts: K "Gain"; tau "Settling time"; Init "Initial input"; T "Sample time"
      mask DialogControl DescGroupVar Prompt: PT1 (IIR)
      mask DialogControl DescTextVar Prompt: IIR form of a PT1 filter
      mask Display:
      | text(0.5,0.5,get_param(gcb,'K'),'HorizontalAlignment','center','VerticalAlignment','Bottom')
      | text(0.5,0.5,['1 + s*' get_param(gcb,'tau')],'HorizontalAlignment','center','VerticalAlignment','Top')
      | plot([0.3 0.7],[0.5 0.5])
  PT1 as IIR1 : Subsystem  AncestorBlock=FriedrichLibrary/Discrete Stuff/PT1 as IIR  mask{K=1, tau=T1, Init=0, T=Ts_Control}
      mask prompts: K "Gain"; tau "Settling time"; Init "Initial input"; T "Sample time"
      mask DialogControl DescGroupVar Prompt: PT1 (IIR)
      mask DialogControl DescTextVar Prompt: IIR form of a PT1 filter
      mask Display:
      | text(0.5,0.5,get_param(gcb,'K'),'HorizontalAlignment','center','VerticalAlignment','Bottom')
      | text(0.5,0.5,['1 + s*' get_param(gcb,'tau')],'HorizontalAlignment','center','VerticalAlignment','Top')
      | plot([0.3 0.7],[0.5 0.5])
  Sum : Sum  Inputs=-+|
  Sum1 : Sum  Inputs=|+-
  Trigonometric Function : Trigonometry  Operator=sincos
  Unit Delay : UnitDelay  SampleTime=Ts_Control  HasFrameUpgradeWarning=on
  ab0->dq0 SinCos : Subsystem  AncestorBlock=FriedrichLibrary/Transformations/ab0->dq0 SinCos
      mask Display:
      | plot(0,0,1,1)
      | text(0.05,0.8,'\alpha\beta0','texmode','on')
      | text(1,0.5,'dq0','horizontalalignment','right')
      | text(0.05,0.3,'sincos','texmode','on')
  "ab0->dq0 SinCos " : Subsystem  AncestorBlock=FriedrichLibrary/Transformations/ab0->dq0 SinCos
      mask Display:
      | plot(0,0,1,1)
      | text(0.05,0.8,'\alpha\beta0','texmode','on')
      | text(1,0.5,'dq0','horizontalalignment','right')
      | text(0.05,0.3,'sincos','texmode','on')
  dq0->ab0 SinCos : Subsystem  AncestorBlock=FriedrichLibrary/Transformations/dq0->ab0 SinCos
      mask Display:
      | plot(0,0,1,1)
      | text(0.05,0.8,'dq0')
      | text(1,0.5,'\alpha\beta0','texmode','on','horizontalalignment','right')
      | text(0.05,0.3,'sincos','texmode','on')
  "dq0->ab0 SinCos " : Subsystem  AncestorBlock=FriedrichLibrary/Transformations/dq0->ab0 SinCos
      mask Display:
      | plot(0,0,1,1)
      | text(0.05,0.8,'dq0')
      | text(1,0.5,'\alpha\beta0','texmode','on','horizontalalignment','right')
      | text(0.05,0.3,'sincos','texmode','on')
  dq0_PS : Outport  PortDimensions=3  VectorParamsAs1DForOutWhenUnconnected=off
  dq0_NS : Outport  Port=2  PortDimensions=3  VectorParamsAs1DForOutWhenUnconnected=off
  wires:
  Unit Delay/1 -> Sum/1
  PT1 as IIR1/1(Y) -> "ab0->dq0 SinCos "/1(ab0)
  PT1 as IIR/1(Y) -> dq0->ab0 SinCos/1(ab0)
  Sum1/1 -> ab0->dq0 SinCos/1(ab0)
  "ab0->dq0 SinCos "/1(dq0) -> Sum1/2
  Mux/1 -> dq0->ab0 SinCos/2(sincos), ab0->dq0 SinCos/2(sincos), "ab0->dq0 SinCos "/2(sincos), "dq0->ab0 SinCos "/2(sincos)
  Trigonometric Function/2 -> Mux/2
  Trigonometric Function/1 -> Mux/1
  w/1 -> Trigonometric Function/1
  Sum/1 -> "dq0->ab0 SinCos "/1(ab0)
  dq0->ab0 SinCos/1(dq0) -> Unit Delay/1
  ab0->dq0 SinCos/1(dq0) -> dq0_PS/1, PT1 as IIR/1(U)
  ab0/1 -> Sum/2, Sum1/1
  "dq0->ab0 SinCos "/1(dq0) -> dq0_NS/1, PT1 as IIR1/1(U)
